simulink model "UpdatedIRECModel"  (R2025b)
settings: Solver=VariableStepAuto  StartTime=0.0  StopTime=65  MaxStep=0.001  RelTol=1e-3
model workspace (MAT data in the model file):
  bca = Simulink.Parameter
  bca.Value = [1 2]
  bca.Complexity = 'real'
  bca.Dimensions = [1 2]
  bca.DataType = 'auto'
  brakeAngle = Simulink.Parameter
  brakeAngle.Complexity = 'real'
  brakeAngle.Dimensions = [0 0]
  brakeAngle.DataType = 'auto'
undefined symbols (not defined in the file or in its folder): F, Light, MIL
libraries: aerolibanim x1, aerolibwind2 x1, aerolibatmos2 x1, aerolibasang x1
settings Model: PacingRate=141  Creator=noahweiss  LastModifiedBy=lawtonskaling

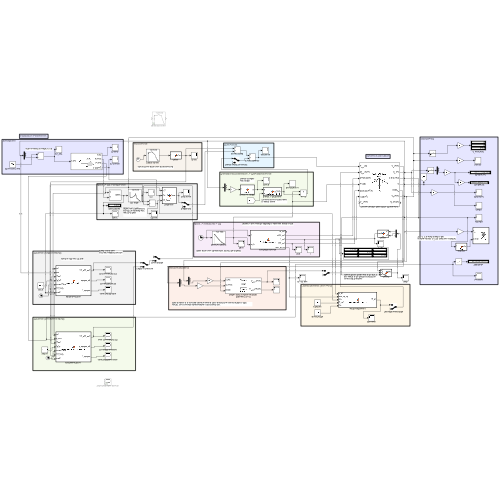
[thumbnail: Simulink's stored preview of the top-level diagram]
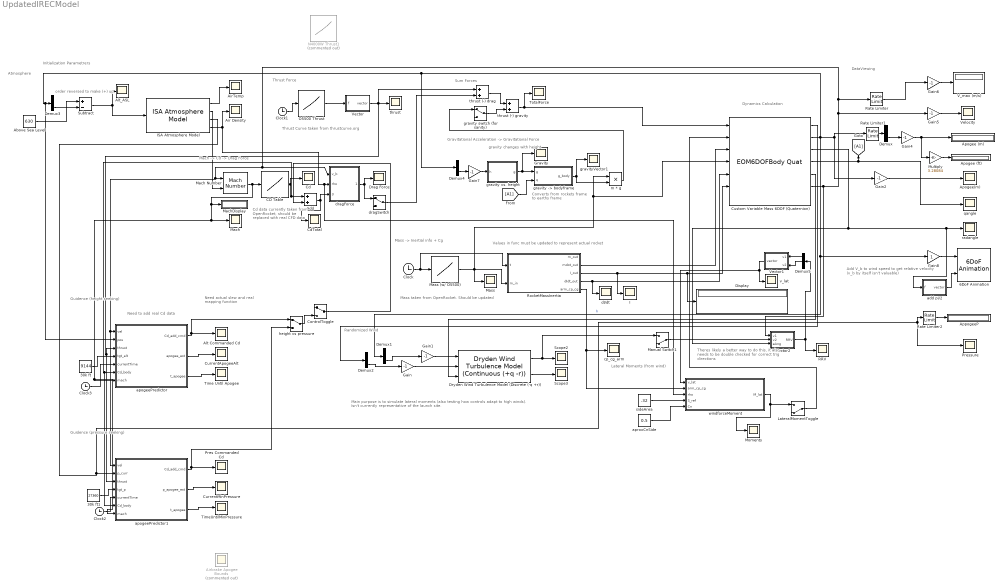
== system UpdatedIRECModel ==
  note: Theres likely a better way to do this, it also needs to be double checked for correct trig directions
  note: Need actual slew
      | and real mapping function
  note: Need to add real Cd data
  note: Guidence (height seeking)
  note: Add V_b to wind speed to get
      | relative velocity (v_b by itself isn't valuable)
  note: Values in func must be updated to represent actual rocket
  note: Lateral Moments (from wind)
  note: Main purpose is to simulate lateral moments (also testing how controls adapt to high winds). Isn't currently representative of the launch site.
  note: Randomized Wind
  note: Converts from rockets frame
      | to earths frame
  note: gravity changes
      | with height
  note: Gravitational Acceleration -> Gravitational Force
  note: Mass taken from OpenRocket. Should be updated
  note: Mass -> Inertial info + Cg
  note: Sum Forces
  note: Thrust Curve taken from thrustcurve.org
  note: Thrust Force
  note: Cd data currently
      | taken from OpenRocket, should be replaced with real CFD data
  note: Mach -> Cd -> Drag Force
  note: order reversed to make (+) up
  note: Atmosphere
  note: Initialization Parametrers
  note: Dynamics Calculation
  note: DataViewing
  note: Guidence (pressure seeking)
  30k ft : Constant  Value=9144
  30k ft1 : Constant  Value=27360
  6DoF Animation : aerolibanim/6DoF Animation  u1=[-1000 1000 -1000 1000 -10000 0]  u2=0.1  u3=200  u4=[4000 0 -5000]  u5=Fixed position  u6=[4000 -4000 -200]  u7=10  u8=off
  Above Sea Level : Constant  Value=630
  Add : Sum
  Air Density : Scope
      settings: ActiveDisplayYMinimum=0.32836250442397086  ActiveDisplayYMaximum=1.3513391175478189  DataLoggingVariableName=ScopeData2
  AirTemp : Scope
      settings: ActiveDisplayYMinimum=208.39933334266343  ActiveDisplayYMaximum=294.3971353024794  DataLoggingVariableName=ScopeData5
  "Airbrake Apogee Bounds " : Scope  Commented=on  NumInputPorts=3
      settings: DataLoggingVariableName=ScopeData31
  Alt Commanded Cd : Scope
      settings: ActiveDisplayYMinimum=-0.21249999999999994  ActiveDisplayYMaximum=1.9124999999999999  DataLoggingVariableName=ScopeData23
  Alt_ASL : Scope
      settings: ActiveDisplayYMinimum=-1  ActiveDisplayYMaximum=1  DataLoggingVariableName=ScopeData15
  Apogee (ft) : Display
  Apogee (m) : Display
      settings: Decimation=4
  Apogee(m) : Scope
      settings: ActiveDisplayYMinimum=-3110.5103645307609  ActiveDisplayYMaximum=11354.709569858003
  AppogeeP : Display
      settings: Decimation=4
  CD Table : Lookup_n-D  NumberOfTableDimensions=1  BreakpointsForDimension1=[0.007, 0.008, 0.01, 0.013, 0.017, 0.024, 0.03, 0.033, 0.037, 0.042, 0.048, 0.051, 0.056, 0.061, 0.067, 0.074, 0.08, 0.086, 0.092, 0.098, 0.102, 0.108, 0.114, 0.12, 0.126, 0.132, 0.138, 0.147, 0.161, 0.182, 0.198, 0.221, 0.248, 0.282, 0.316, 0.34, 0.375, 0.41, 0.432, 0.465, 0.502, 0.538, 0.575, 0.612, 0.647, 0.685, 0.723, 0.76, 0.798, 0.837, 0.858, 0.89, 0.929, 0.968, 1.007, 1.033, 1.071, 1.103, 1.141, 1.149, 1.16, 1.177, 1.182, 1.188, 1.197, 1.206, 1.219, 1.238, 1.257, 1.285, 1.32, 1.356, 1.368, 1.386, 1.413, 1.447, 1.48, 1.504, 1.536, 1.569, 1.601, 1.632, 1.664, 1.695, 1.725, 1.727, 1.73, 1.734, 1.74, 1.75, 1.763, 1.784, 1.793, 1.806, 1.826, 1.852, 1.876, 1.897, 1.917, 1.934, 1.937, 1.942, 1.95, 1.961, 1.969, 1.979, 1.992, 1.999, 2.008, 2.018, 2.026, 2.029, 2.033, 2.037, 2.038, 2.039, 2.041, 2.042, 2.044, 2.045, 2.046]  Table=[0.463, 0.452, 0.425, 0.409, 0.389, 0.367, 0.354, 0.348, 0.341, 0.339, 0.339, 0.339, 0.339, 0.339, 0.339, 0.339, 0.339, 0.339, 0.339, 0.339, 0.339, 0.34, 0.34, 0.34, 0.34, 0.34, 0.34, 0.34, 0.34, 0.34, 0.34, 0.341, 0.341, 0.342, 0.342, 0.343, 0.344, 0.344, 0.345, 0.346, 0.347, 0.349, 0.35, 0.352, 0.354, 0.356, 0.359, 0.362, 0.366, 0.372, 0.375, 0.383, 0.382, 0.377, 0.381, 0.408, 0.427, 0.426, 0.413, 0.409, 0.403, 0.392, 0.389, 0.385, 0.379, 0.373, 0.364, 0.352, 0.342, 0.331, 0.325, 0.321, 0.32, 0.318, 0.315, 0.311, 0.307, 0.305, 0.301, 0.298, 0.294, 0.291, 0.288, 0.285, 0.282, 0.281, 0.281, 0.281, 0.28, 0.279, 0.278, 0.276, 0.275, 0.274, 0.272, 0.269, 0.267, 0.265, 0.263, 0.262, 0.262, 0.261, 0.26, 0.259, 0.259, 0.258, 0.257, 0.256, 0.255, 0.254, 0.254, 0.253, 0.253, 0.253, 0.253, 0.252, 0.252, 0.252, 0.252, 0.252, 0.252]  InternalRulePriority=Speed  RndMeth=Simplest
  Cd : Scope
      settings: ActiveDisplayYMinimum=-0.14855998025047912  ActiveDisplayYMaximum=1.8026279606623583  DataLoggingVariableName=ScopeData8
  CdTotal : Scope
      settings: ActiveDisplayYMinimum=-0.16752402901527019  ActiveDisplayYMaximum=2.158206654782723  DataLoggingVariableName=ScopeData20
  Clock{,1..3} (4 alike) : Clock
  ControlToggle : ManualSwitch
  CurrentApogeeAlt : Scope
      settings: ActiveDisplayYMinimum=-1288.6434664799376  ActiveDisplayYMaximum=11597.791198319441  DataLoggingVariableName=ScopeData24
  CurrentMinPressure : Scope
      settings: ActiveDisplayYMinimum=22558.660012318163  ActiveDisplayYMaximum=101918.03026412864  DataLoggingVariableName=ScopeData22
  Custom Variable Mass 6DOF (Quaternion) : EOM6DOFBodyQuat  mtype=Custom Variable  vre_flag=on
  Demux{,1..5} (6 alike) : Demux  Outputs=3
  Display : Display
  Drag Force : Scope
      settings: ActiveDisplayYMinimum=-997.38496868055154  ActiveDisplayYMaximum=2083.9665587051204  DataLoggingVariableName=ScopeData3
  Dryden Wind Turbulence Model (Discrete (-q +r)) : aerolibwind2/Dryden Wind Turbulence Model  (Continuous (+q -r))  units=Metric (MKS)  spec=MIL-F-8785C  model=Discrete Dryden (+q +r)  W20=5  Wdeg=0  TurbProb=10^-2 - Light  L_high=533.4  Wingspan=1  ts=0.1  Seed=[23341 23342 23343 23345]  T_on=on
      settings: LibrarySourceBlock=|
      | aerolibwind2/Dryden Wind Turbulence Model
      | (Discrete (-q +r))
  Gain{,1..2,4..7} (7 alike) : Gain  Gain=-1
  Gain8 : Gain
  Gravity : Scope
      settings: ActiveDisplayYMinimum=9.68035453491508  ActiveDisplayYMaximum=9.8834339095755688  DataLoggingVariableName=ScopeData9
  I : Scope
      settings: ActiveDisplayYMinimum=-2.0972210212356206  ActiveDisplayYMaximum=8.771099345696328  DataLoggingVariableName=ScopeData12
  ISA Atmosphere Model : aerolibatmos2/ISA Atmosphere Model  useExtended=off  action=None  custom=off  viscosityOut=off  g=9.80665  gamma=1.4  R=287.0531  L=0.0065  h_trop=11000  h_strat=20000  rho0=1.225  P0=101325  T0=288.15  h0=0  S=110.4  Tref=273.15  muref=1.716e-5
  LateralMomentToggle : ManualSwitch  CurrentSetting=0
  Mach : Scope
      settings: ActiveDisplayYMinimum=-0.28015884352453835  ActiveDisplayYMaximum=2.052851576354866  DataLoggingVariableName=ScopeData4
  Mach Number : aerolibasang/Mach Number
  MachDisplay : Display
  Manual Switch1 : ManualSwitch  CurrentSetting=0
  Mass : Scope
      settings: ActiveDisplayYMinimum=17.378289742266098  ActiveDisplayYMaximum=34.057183726794406  DataLoggingVariableName=ScopeData7
  Mass (w/ O5500) : Lookup_n-D  NumberOfTableDimensions=1  BreakpointsForDimension1=[0, 0.009, 0.019, 0.029, 0.039, 0.044, 0.051, 0.063, 0.073, 0.078, 0.086, 0.094, 0.104, 0.109, 0.117, 0.125, 0.135, 0.147, 0.157, 0.167, 0.177, 0.187, 0.194, 0.204, 0.214, 0.224, 0.234, 0.244, 0.254, 0.269, 0.292, 0.325, 0.35, 0.387, 0.428, 0.478, 0.528, 0.563, 0.613, 0.663, 0.694, 0.74, 0.79, 0.84, 0.891, 0.941, 0.988, 1.038, 1.088, 1.138, 1.188, 1.238, 1.266, 1.308, 1.358, 1.408, 1.458, 1.491, 1.541, 1.581, 1.631, 1.641, 1.656, 1.679, 1.684, 1.692, 1.705, 1.716, 1.733, 1.759, 1.784, 1.822, 1.871, 1.921, 1.938, 1.964, 2.003, 2.053, 2.103, 2.138, 2.188, 2.238, 2.288, 2.338, 2.388, 2.438, 2.488, 2.491, 2.496, 2.502, 2.512, 2.528, 2.55, 2.585, 2.6, 2.623, 2.658, 2.708, 2.758, 2.808, 2.858, 2.908, 2.919, 2.935, 2.96, 2.997, 3.022, 3.06, 3.11, 3.138, 3.181, 3.231, 3.281, 3.3, 3.329, 3.373, 3.388, 3.41, 3.441, 3.487, 3.537, 3.544, 3.555, 3.571, 3.595, 3.609, 3.629, 3.66, 3.688, 3.73, 3.778, 3.819]  BreakpointsForDimension1FirstPoint=0  BreakpointsForDimension1Spacing=.05  Table=[31.41, 31.41, 31.39, 31.38, 31.36, 31.35, 31.33, 31.29, 31.26, 31.25, 31.22, 31.2, 31.17, 31.15, 31.13, 31.1, 31.07, 31.04, 31.01, 30.98, 30.95, 30.92, 30.9, 30.86, 30.83, 30.8, 30.77, 30.74, 30.71, 30.67, 30.6, 30.5, 30.42, 30.3, 30.17, 30.01, 29.84, 29.73, 29.56, 29.39, 29.29, 29.13, 28.96, 28.79, 28.62, 28.45, 28.28, 28.11, 27.93, 27.76, 27.59, 27.41, 27.32, 27.17, 26.99, 26.82, 26.64, 26.53, 26.35, 26.21, 26.04, 26.0, 25.95, 25.87, 25.85, 25.83, 25.79, 25.75, 25.69, 25.6, 25.52, 25.4, 25.24, 25.08, 25.03, 24.95, 24.83, 24.68, 24.53, 24.43, 24.29, 24.15, 24.01, 23.87, 23.73, 23.59, 23.45, 23.44, 23.43, 23.41, 23.38, 23.34, 23.28, 23.19, 23.15, 23.1, 23.03, 22.92, 22.82, 22.71, 22.61, 22.5, 22.48, 22.45, 22.41, 22.35, 22.32, 22.26, 22.19, 22.15, 22.1, 22.04, 21.98, 21.96, 21.93, 21.89, 21.88, 21.86, 21.84, 21.81, 21.78, 21.77, 21.77, 21.76, 21.74, 21.73, 21.72, 21.71, 21.69, 21.68, 21.66, 21.65]  ExtrapMethod=Clip  UseLastTableValue=on  InternalRulePriority=Speed  RndMeth=Simplest  SupportTunableSize=on
  Moments : Scope
      settings: ActiveDisplayYMinimum=-0.037322938130257846  ActiveDisplayYMaximum=0.019814293763566297  DataLoggingVariableName=ScopeData19
  Multiply : Gain  Gain=3.28084
  N4000W Thrust1 : Lookup_n-D  Commented=on  NumberOfTableDimensions=1  BreakpointsForDimension1=[0.01;0.029;0.03;0.031;0.039;0.049;0.05;0.06;0.07000000000000001;0.078;0.08799999999999999;0.12;0.148;0.247;0.398;0.577;0.774;0.964;1.172;1.341;1.51;1.661;1.837;2.027;2.157;2.295;2.336;2.505;2.633;2.794;2.97;3.131;3.3;3.449;3.547;3.607;3.708;3.825;3.927;4.054;4.205;4.314;4.394;4.462;4.511;4.631;4.761;4.854;4.906]  Table=[39.369999999999997;393.70100000000002;1742.126;2209.6460000000002;2874.0160000000001;2534.4490000000001;3469.4879999999998;3809.0549999999998;4079.7240000000002;4242.1260000000002;4384.8429999999998;4330.7089999999998;4227.3620000000001;4242.1260000000002;4296.2600000000002;4350.3940000000002;4438.9759999999997;4512.7950000000001;4566.9290000000001;4621.0630000000001;4621.0630000000001;4655.5119999999997;4675.1970000000001;4709.6459999999997;4729.3310000000001;4749.0159999999996;4749.0159999999996;4694.8819999999996;4655.5119999999997;4547.2439999999997;4478.3459999999995;4384.8429999999998;4315.9449999999997;4261.8109999999997;4261.8109999999997;4207.6769999999997;3720.4720000000002;2893.701;2445.866;2155.5120000000002;1850.394;1471.4570000000001;1097.441;841.53499999999997;698.81899999999996;521.654;265.74799999999999;123.03100000000001;0]  ExtrapMethod=Clip  UseLastTableValue=on  InternalRulePriority=Speed  RndMeth=Simplest
  O5500 Thrust : Lookup_n-D  NumberOfTableDimensions=1  BreakpointsForDimension1=[0.009, 0.044, 0.063, 0.078, 0.094, 0.109, 0.125, 0.147, 0.194, 0.35, 0.428, 0.563, 0.694, 0.988, 1.266, 1.491, 1.581, 1.641, 1.684, 1.716, 1.784, 1.938, 2.138, 2.491, 2.6, 2.919, 3.022, 3.138, 3.3, 3.388, 3.441, 3.544, 3.609, 3.688, 3.778, 3.819, 3.853, 3.897, 3.981, 3.997]  Table=[20.408, 7112.245, 6734.694, 6897.959, 6612.245, 6765.306, 6540.816, 6581.633, 6520.408, 6795.918, 7091.837, 7285.714, 7408.163, 7581.633, 7622.449, 7724.49, 7653.061, 7540.816, 7500.0, 7336.735, 7224.49, 6785.714, 6326.531, 5897.959, 5704.082, 3540.816, 3408.163, 2887.755, 2234.694, 1673.469, 1489.796, 1418.367, 1295.918, 816.327, 653.061, 581.633, 489.796, 285.714, 20.408, 0.0]  ExtrapMethod=Clip  UseLastTableValue=on  InternalRulePriority=Speed  RndMeth=Simplest
  Pres Commanded Cd : Scope
      settings: ActiveDisplayYMinimum=-0.13333983055562462  ActiveDisplayYMaximum=1.2000584750006218  DataLoggingVariableName=ScopeData27
  Pressure : Scope
      settings: ActiveDisplayYMinimum=27434.677675772422  ActiveDisplayYMaximum=27734.888035030621  DataLoggingVariableName=ScopeData28
  RRV : Scope
      settings: ActiveDisplayYMinimum=-147.82773037596519  ActiveDisplayYMaximum=87.725846488197178  DataLoggingVariableName=ScopeData30
  Rate Limiter : RateLimiter  RisingSlewLimit=0  FallingSlewLimit=-99999  SampleTimeMode=inherited
  Rate Limiter1 : RateLimiter  RisingSlewLimit=0  FallingSlewLimit=-99999  SampleTimeMode=inherited
  Rate Limiter2 : RateLimiter  RisingSlewLimit=0  FallingSlewLimit=-99999  SampleTimeMode=inherited
  RocketMassInertia : MATLAB Function  TreatAsAtomicUnit=on
  Scope2 : Scope
      settings: ActiveDisplayYMinimum=-3.5919608640744958  ActiveDisplayYMaximum=4.9299230789313464  DataLoggingVariableName=ScopeData10
  Scope3 : Scope
      settings: ActiveDisplayYMinimum=-6.9396586411031267E+307  ActiveDisplayYMaximum=1.2409351060971885E+307  DataLoggingVariableName=ScopeData13
  Subtract : Sum  Inputs=+-
  Time Until Apogee : Scope
      settings: ActiveDisplayYMinimum=-142.04754177762925  ActiveDisplayYMaximum=334.02527575200287  DataLoggingVariableName=ScopeData25
  "TimeUntilMinPressure " : Scope
      settings: ActiveDisplayYMinimum=-169.43788860496815  ActiveDisplayYMaximum=400.46442472293245  DataLoggingVariableName=ScopeData26
  TotalForce : Scope
      settings: ActiveDisplayYMinimum=-1336.7372091363745  ActiveDisplayYMaximum=2383.8615158167772  DataLoggingVariableName=ScopeData6
  V_max (m/s) : Display
  Vector : MATLAB Function  TreatAsAtomicUnit=on
  Vector1 : MATLAB Function  TreatAsAtomicUnit=on
  Vector2 : MATLAB Function  TreatAsAtomicUnit=on
  Velocity : Scope
      settings: ActiveDisplayYMinimum=-269.31086851436129  ActiveDisplayYMaximum=736.30958702242276
  add pi/2 : MATLAB Function  TreatAsAtomicUnit=on
  apogeePredictor : MATLAB Function  TreatAsAtomicUnit=on
  apogeePredictor1 : MATLAB Function  TreatAsAtomicUnit=on
  aproxCnSide : Constant  Value=0.5
  cp_cg_arm : Scope
      settings: ActiveDisplayYMinimum=-0.50903350176661866  ActiveDisplayYMaximum=0.54777232101906159  DataLoggingVariableName=ScopeData21
  dI/dt : Scope
      settings: ActiveDisplayYMinimum=-1  ActiveDisplayYMaximum=1  DataLoggingVariableName=ScopeData11
  dragForce : MATLAB Function  TreatAsAtomicUnit=on
  dragSwitch : ManualSwitch
  "gravity -> bodyframe" : MATLAB Function  TreatAsAtomicUnit=on
  gravity switch (for sanity) : ManualSwitch
  gravity vs. height : MATLAB Function  TreatAsAtomicUnit=on
  gravityVector1 : Scope
      settings: ActiveDisplayYMinimum=-243.141573178529  ActiveDisplayYMaximum=145.53469052356505  DataLoggingVariableName=ScopeData17
  height vs pressure : ManualSwitch
  m * g : Product
  qangle : Scope
      settings: ActiveDisplayYMinimum=-0.69920344245396326  ActiveDisplayYMaximum=1.5743399638672304  DataLoggingVariableName=ScopeData18
  radangle : Scope
      settings: ActiveDisplayYMinimum=-3.9268979901815744  ActiveDisplayYMaximum=3.926971640420561  DataLoggingVariableName=ScopeData16
  sideArea : Constant  Value=.32
  thrust : Scope
      settings: ActiveDisplayYMinimum=-6112.1844862335238  ActiveDisplayYMaximum=743.283877041516  DataLoggingVariableName=ScopeData14
  thrust (-) drag : Sum
  thrust (-) gravity : Sum
  v_lat : Scope
      settings: ActiveDisplayYMinimum=-11.656849883026286  ActiveDisplayYMaximum=6.4269462139654019  DataLoggingVariableName=ScopeData29
  windforceMoment : MATLAB Function  TreatAsAtomicUnit=on
  wires:
  Custom Variable Mass 6DOF (Quaternion)/6 -> Vector2/1(v1), dragForce/1(v_b), apogeePredictor1/1(vel), apogeePredictor/1(vel), Mach Number/1, Rate Limiter/1, Gain5/1
  Rate Limiter/1 -> Gain6/1
  ISA Atmosphere Model/4 -> windforceMoment/3(rho), dragForce/2(rho), Air Density/1
  Rate Limiter1/1 -> Demux/1
  Demux/3 -> Gain4/1
  dragForce/1(drag_force) -> Drag Force/1, dragSwitch/1
  CD Table/1 -> apogeePredictor1/6(Cd_body), apogeePredictor/6(Cd_body), Add/1, Cd/1
  ISA Atmosphere Model/1 -> AirTemp/1
  Clock1/1 -> O5500 Thrust/1
  O5500 Thrust/1 -> Vector/1(f)
  Vector/1(vector) -> thrust (-) drag/1, apogeePredictor1/3(thrust), apogeePredictor/3(thrust), thrust/1
  dragSwitch/1 -> thrust (-) drag/2
  RocketMassInertia/4(dIdt_out) -> Custom Variable Mass 6DOF (Quaternion)/5, dI/dt/1
  RocketMassInertia/3(I_out) -> I/1, Custom Variable Mass 6DOF (Quaternion)/6, Display/1
  Mass (w/ O5500)/1 -> RocketMassInertia/2(m_in), Custom Variable Mass 6DOF (Quaternion)/4, m * g/1, Mass/1
  thrust (-) drag/1 -> thrust (-) gravity/1
  thrust (-) gravity/1 -> Custom Variable Mass 6DOF (Quaternion)/1, TotalForce/1
  m * g/1 -> gravity switch (for sanity)/1
  gravity switch (for sanity)/1 -> thrust (-) gravity/2
  Above Sea Level/1 -> Subtract/1
  Custom Variable Mass 6DOF (Quaternion)/2 -> Gain2/1, Rate Limiter1/1, Gain8/1, Demux1/1, Demux4/1, apogeePredictor/2(pos), Demux3/1  "h"
  "gravity -> bodyframe"/1(g_body) -> gravityVector1/1, m * g/2
  Custom Variable Mass 6DOF (Quaternion)/5 -> Dryden Wind Turbulence Model (Discrete (-q +r))/3
  Dryden Wind Turbulence Model (Discrete (-q +r))/1 -> Scope2/1, Manual Switch1/1
  Dryden Wind Turbulence Model (Discrete (-q +r))/2 -> Scope3/1
  Demux1/3 -> Gain1/1
  Demux2/3 -> Gain/1
  Custom Variable Mass 6DOF (Quaternion)/1 -> Demux2/1
  Gain/1 -> Dryden Wind Turbulence Model (Discrete (-q +r))/2
  Gain1/1 -> Dryden Wind Turbulence Model (Discrete (-q +r))/1
  RocketMassInertia/2(mdot_out) -> Custom Variable Mass 6DOF (Quaternion)/3
  Custom Variable Mass 6DOF (Quaternion)/3 -> add pi/2/1(f), radangle/1, Vector2/3(eAng)
  Manual Switch1/1 -> Vector2/2(v2)
  Demux3/3 -> Subtract/2
  Subtract/1 -> ISA Atmosphere Model/1, Alt_ASL/1
  ISA Atmosphere Model/2 -> Mach Number/2
  Mach Number/1 -> Mach/1, apogeePredictor1/7(mach), apogeePredictor/7(mach), MachDisplay/1, CD Table/1
  Gain2/1 -> Apogee(m)/1
  Gain5/1 -> Velocity/1
  Gain6/1 -> V_max (m/s)/1
  Gain4/1 -> Multiply/1, Apogee (m)/1
  gravity vs. height/1(g) -> Gravity/1, "gravity -> bodyframe"/1(g)
  Gain7/1 -> gravity vs. height/1(h)
  Demux4/3 -> Gain7/1
  Custom Variable Mass 6DOF (Quaternion)/4 -> qangle/1, [A1]
  aproxCnSide/1 -> windforceMoment/5(Cn)
  LateralMomentToggle/1 -> Custom Variable Mass 6DOF (Quaternion)/2
  sideArea/1 -> windforceMoment/4(S_ref)
  Gain8/1 -> 6DoF Animation/1
  [A1] -> "gravity -> bodyframe"/2(q)
  Clock/1 -> RocketMassInertia/1(t), Mass (w/ O5500)/1
  Multiply/1 -> Apogee (ft)/1
  windforceMoment/1(M_lat) -> Moments/1, LateralMomentToggle/1
  30k ft/1 -> apogeePredictor/4(tgt_alt)
  Clock3/1 -> apogeePredictor/5(currentTime)
  apogeePredictor/2(apogee_est) -> CurrentApogeeAlt/1
  apogeePredictor/3(t_apogee) -> Time Until Apogee/1
  RocketMassInertia/5(arm_cp_cg) -> windforceMoment/2(arm_cp_cg), cp_cg_arm/1
  apogeePredictor/1(Cd_add_cmd) -> height vs pressure/1, Alt Commanded Cd/1
  Add/1 -> CdTotal/1, dragForce/3(Cd_base)
  ControlToggle/1 -> Add/2
  add pi/2/1(vector) -> 6DoF Animation/2
  apogeePredictor1/3(t_apogee) -> "TimeUntilMinPressure "/1
  apogeePredictor1/1(Cd_add_cmd) -> height vs pressure/2, Pres Commanded Cd/1
  apogeePredictor1/2(p_apogee_est) -> CurrentMinPressure/1
  30k ft1/1 -> apogeePredictor1/4(tgt_p)
  Clock2/1 -> apogeePredictor1/5(currentTime)
  height vs pressure/1 -> ControlToggle/2
  ISA Atmosphere Model/3 -> Rate Limiter2/1, Pressure/1, apogeePredictor1/2(p_curr)
  Rate Limiter2/1 -> AppogeeP/1
  Vector1/1(vector) -> windforceMoment/1(v_lat), v_lat/1
  Demux5/1 -> Vector1/1(v1)
  Demux5/2 -> Vector1/2(v2)
  Vector2/1(RRV) -> RRV/1, Demux5/1

== matlab function UpdatedIRECModel/Vector1 ==
  data: v1 input; v2 input; vector output
function vector = fcn(v1, v2)

vector = zeros(1,3);
vector(1) = v1;
vector(2) = v2;

end

== matlab function UpdatedIRECModel/Vector2 ==
  data: v1 input; v2 input; RRV output; eAng input
function RRV = fcn(v1, v2, eAng)

RRV = zeros(1,3);
RRV(1) = v1(1) + cos(eAng(1)) * v2(1);
RRV(2) = v1(2) + cos(eAng(2)) * v2(2);
RRV(3) = v1(3) + cos(eAng(3)) * v2(3);

end

== matlab function UpdatedIRECModel/RocketMassInertia ==
  settings: updateMethod=DISCRETE
  data: t input; m_out output; mdot_out output; I_out output; dIdt_out output; m_in input; arm_cp_cg output
function [m_out, mdot_out, I_out, dIdt_out, arm_cp_cg] = RocketMassInertia(t, m_in)

persistent m0_total m_prop0

D_body   = 0.1016;
R_body   = D_body/2;

L_total  = 2.40;
L_nose   = 0.45;
L_body   = L_total - L_nose;

L_motor     = 0.65;
x_motor_fwd = L_total - L_motor;
x_motor_aft = L_total;

x_nose_cg   = 0.27 * L_nose;
x_tube_cg   = L_nose + 0.5 * L_body;
x_avionics  = L_nose + 0.15;
x_airbrake  = L_nose + 0.90;
x_fins      = L_total - 0.05;
x_case      = x_motor_fwd + 0.5 * L_motor;
x_other     = x_avionics;

m_nose     = 0.8;
m_tube     = 1.2;
m_avionics = 0.7;
m_airbrake = 0.5;
m_case     = 1.0;
m_fins     = 0.6;
m_other    = 0.4;

m_struct_total = m_nose + m_tube + m_avionics + m_airbrake + m_case + m_fins + m_other;

R_prop  = 0.035;

if isempty(m0_total)
    m0_total = m_in;
    m_prop0  = max(m0_total - m_struct_total, 0);
end

m_total = m_in;
if m_total < m_struct_total
    m_total = m_struct_total;
end

m_prop = m_total - m_struct_total;
if m_prop < 0
    m_prop = 0;
end
if m_prop > m_prop0
    m_prop = m_prop0;
end

x_prop_cg = x_case;
L_prop    = L_motor;

Ixx_tube_cg = 0.5 * m_tube * R_body^2;
Iyy_tube_cg = m_tube * (L_body^2 / 12 + R_body^2 / 4);
Izz_tube_cg = Iyy_tube_cg;

if m_prop > 0
    Ixx_prop_cg = 0.5 * m_prop * R_prop^2;
    Iyy_prop_cg = m_prop * (L_prop^2 / 12 + R_prop^2 / 4);
    Izz_prop_cg = Iyy_prop_cg;
else
    Ixx_prop_cg = 0;
    Iyy_prop_cg = 0;
    Izz_prop_cg = 0;
end

Ixx_case_cg = 0.5 * m_case * R_prop^2;
Iyy_case_cg = m_case * (L_motor^2 / 12 + R_prop^2 / 4);
Izz_case_cg = Iyy_case_cg;

m_total_components = m_struct_total + m_prop;

if m_total_components <= 0
    x_cg = x_tube_cg;
else
    x_cg = (m_nose * x_nose_cg + m_tube * x_tube_cg + m_avionics * x_avionics + ...
            m_airbrake * x_airbrake + m_case * x_case + m_fins * x_fins + ...
            m_other * x_other + m_prop * x_prop_cg) / m_total_components;
end

dx_tube  = x_tube_cg   - x_cg;
dx_case  = x_case      - x_cg;
dx_prop  = x_prop_cg   - x_cg;
dx_nose  = x_nose_cg   - x_cg;
dx_av    = x_avionics  - x_cg;
dx_ab    = x_airbrake  - x_cg;
dx_fin   = x_fins      - x_cg;
dx_other = x_other     - x_cg;

Ixx_tube = Ixx_tube_cg;
Iyy_tube = Iyy_tube_cg + m_tube     * dx_tube^2;
Izz_tube = Izz_tube_cg + m_tube     * dx_tube^2;

Ixx_case = Ixx_case_cg;
Iyy_case = Iyy_case_cg + m_case     * dx_case^2;
Izz_case = Izz_case_cg + m_case     * dx_case^2;

Ixx_prop = Ixx_prop_cg;
Iyy_prop = Iyy_prop_cg + m_prop     * dx_prop^2;
Izz_prop = Izz_prop_cg + m_prop     * dx_prop^2;

Ixx_nose = 0;
Iyy_nose = m_nose     * dx_nose^2;
Izz_nose = m_nose     * dx_nose^2;

Ixx_av   = 0;
Iyy_av   = m_avionics * dx_av^2;
Izz_av   = m_avionics * dx_av^2;

Ixx_ab   = 0;
Iyy_ab   = m_airbrake * dx_ab^2;
Izz_ab   = m_airbrake * dx_ab^2;

Ixx_fin  = 0;
Iyy_fin  = m_fins     * dx_fin^2;
Izz_fin  = m_fins     * dx_fin^2;

Ixx_other = 0;
Iyy_other = m_other   * dx_other^2;
Izz_other = m_other   * dx_other^2;

Ixx = Ixx_tube + Ixx_case + Ixx_prop + Ixx_nose + Ixx_av + Ixx_ab + Ixx_fin + Ixx_other;
Iyy = Iyy_tube + Iyy_case + Iyy_prop + Iyy_nose + Iyy_av + Iyy_ab + Iyy_fin + Iyy_other;
Izz = Izz_tube + Izz_case + Izz_prop + Izz_nose + Izz_av + Izz_ab + Izz_fin + Izz_other;

% kill roll coupling: make Iyy = Izz
I_perp = 0.5 * (Iyy + Izz);
Iyy    = I_perp;
Izz    = I_perp;

I_mat = zeros(3,3);
I_mat(1,1) = Ixx;
I_mat(2,2) = Iyy;
I_mat(3,3) = Izz;

m_out    = m_total;
I_out    = I_mat;
dIdt_out = zeros(3,3);
mdot_out = 0;

x_cp = 1.8; % [m] CP from nose (tune this)
arm_cp_cg = x_cp - x_cg;
end

== matlab function UpdatedIRECModel/dragForce ==
  data: v_b input; drag_force output; rho input; Cd_base input
function drag_force = fcn(v_b, rho, Cd_base)

    D = 0.15672;
    R = D/2;
    A_ref = pi * R^2;

    if ~isfinite(rho) || rho <= 0 || ~isfinite(Cd_base) || Cd_base <= 0
        drag_force = zeros(3,1);
        return;
    end

    vx = v_b(1); vy = v_b(2); vz = v_b(3);
    v2 = vx*vx + vy*vy + vz*vz;
    if v2 < 1e-8
        drag_force = zeros(3,1);
        return;
    end

    V = sqrt(v2);
    q = 0.5 * rho * v2;

    % angle of attack relative to body x
    alpha = atan2(sqrt(vy*vy + vz*vz), vx);

    % constrict AoA
    alpha_max = deg2rad(5);       % 5 deg cap
    if alpha > alpha_max
        alpha = alpha_max;
    end

    k_alpha = 0.5;                 % tweak 0–1 range
    Cd_eff = Cd_base + k_alpha * (alpha * alpha);

    Dmag = q * Cd_eff * A_ref;

    drag_force = -(Dmag / V) * v_b;
end

== matlab function UpdatedIRECModel/gravity vs. height ==
  data: h input; g output
function g = gravity(h)

G = 6.674e-11;
M = 5.972e24;
R = 6.371e6;

g = G * M ./ (R + h).^2;
end

== matlab function UpdatedIRECModel/add pi//2 ==
  data: f input; vector output
function vector = fcn(f)
f = f(:);
vector = f;
vector(2) = f(2) + pi/2;
end

== matlab function UpdatedIRECModel/windforceMoment ==
  data: v_lat input; M_lat output; arm_cp_cg input; rho input; S_ref input; Cn input
function M_lat = lateralAeroMoments(v_lat, arm_cp_cg, rho, S_ref, Cn)
   Vx = v_lat(1);
   Vy = v_lat(2);

   if ~isfinite(Vx) || ~isfinite(Vy) || ~isfinite(arm_cp_cg) || ~isfinite(rho) || ~isfinite(S_ref) || ~isfinite(Cn)
        M_lat = [0; 0; 0];
        return;
   end
    
   V_lat = sqrt(Vx*Vx + Vy*Vy);
   q_dyn = 0.5 * rho * (Vx*Vx + Vy*Vy);
   Fn = q_dyn * S_ref * Cn;

   Fx = -Fn * (Vx / V_lat);
   Fy = -Fn * (Vy / V_lat);

   Mx = abs(arm_cp_cg) * Fx;
   My = abs(arm_cp_cg) * Fy;

   M_lat = [Mx; My; 0];

end

== matlab function UpdatedIRECModel/gravity -> bodyframe ==
  data: g input; g_body output; q input
function g_body = gravityBodyQuat(g, q)

q0 = q(1);
q1 = q(2);
q2 = q(3);
q3 = q(4);

% Direction Cosine Matrix: inertial -> body
R = [ 1-2*(q2^2+q3^2),   2*(q1*q2+q0*q3),   2*(q1*q3-q0*q2);
      2*(q1*q2-q0*q3),   1-2*(q1^2+q3^2),   2*(q2*q3+q0*q1);
      2*(q1*q3+q0*q2),   2*(q2*q3-q0*q1),   1-2*(q1^2+q2^2) ];

% Gravity direction in inertial frame (NED)
g_inertial = [0; 0; g];   % +Z = down

% Transform to BODY frame
g_body = R * g_inertial;
end

== matlab function UpdatedIRECModel/Vector ==
  data: f input; vector output
function vector = fcn(f)

vector = zeros(3,1);
vector(3) = -f;

end

== matlab function UpdatedIRECModel/apogeePredictor ==
  settings: updateMethod=DISCRETE
  data: vel input; pos input; thrust input; Cd_add_cmd output; tgt_alt input; currentTime input; apogee_est output; t_apogee output; Cd_body input; mach input
function [Cd_add_cmd, apogee_est, t_apogee] = apogeePredictor(vel, pos, thrust, tgt_alt, currentTime, Cd_body, mach)
    % --- Configuration and Physical Constants ---
    persistent Cd_add_prev t_prev apogee_time prev_vel_up
    m = 18.9;                       % Rocket mass (kg)
    A = 8107/(1000^2);              % Reference area (m^2)
    A_over_m = A/m;
    g0 = 9.80665;                   % Standard gravity
    Re = 6371000;                   % Earth radius
    Cd_body_nominal = 0.7;          % Default dry rocket drag coefficient
    Cd_total_max = 1.7;             % Maximum drag with airbrakes fully deployed
    
    % --- Input Validation and Bounds Handling ---
    if nargin < 6 || isempty(Cd_body)
        Cd_body = Cd_body_nominal;
    end
    if nargin < 7 || isempty(mach)
        mach = 0;
    end
    Cd_body = max(0, Cd_body);
    Cd_air_min = 0;
    Cd_air_max = max(0, Cd_total_max - Cd_body); % Max allowable drag from airbrakes
    
    % --- Control Parameters ---
    burn_window = 3.0;              % Time window for motor burn
    thrust_thresh = 1.0;            % Newton threshold for motor activity
    alt_tol = 0.0;                  % Target altitude tolerance
    max_iter = 12;                  % Iterations for binary search of Cd
    max_rate = 1.5;                 % Max slew rate (Cd change per second)

    % --- Persistent State Initialization ---
    if isempty(Cd_add_prev)
        Cd_add_prev = 0;
    end
    if isempty(t_prev)
        t_prev = currentTime;
    end
    if isempty(apogee_time)
        apogee_time = NaN;
    end
    if isempty(prev_vel_up)
        prev_vel_up = 0;
    end
    
    % --- Timing and Delta-T Calculation ---
    dt_cmd = currentTime - t_prev;
    if dt_cmd <= 0
        dt_cmd = 0.02;
    elseif dt_cmd > 0.1
        dt_cmd = 0.1;
    end
    t_prev = currentTime;
    Cd_add_prev = max(Cd_air_min, min(Cd_air_max, Cd_add_prev));
    
    % --- Coordinate System Mapping ---
    % Identifies the vertical axis based on the largest positional component (assuming ENU/NED)
    if numel(pos) >= 3
        [~, idx] = max([abs(pos(2)), abs(pos(3))]);
        vert_idx = idx + 1;
    else
        vert_idx = 2;
    end
    alt_up = max(0, -pos(vert_idx));  % Conversion to up-positive altitude
    vel_up = -vel(vert_idx);          % Conversion to up-positive velocity
    thrust_mag = norm(thrust);
    
    % --- Apogee Detection ---
    % Monitors for the zero-crossing of vertical velocity
    if isnan(apogee_time)
        if prev_vel_up > 0 && vel_up <= 0
            apogee_time = currentTime;
        end
    end
    prev_vel_up = vel_up;
    
    % --- Default Prediction State ---
    Cd_add_target = Cd_add_prev;  
    apogee_est = alt_up;
    t_apogee = currentTime;
    
    % --- Control Logic State Machine ---
    
    % Case 1: Recovery Phase (Post-apogee)
    if ~isnan(apogee_time) && currentTime >= apogee_time + 2
        Cd_add_target = 0; % Retract airbrakes for parachute deployment
        apogee_est = alt_up;
        t_apogee = apogee_time;
        
    % Case 2: Boost Phase
    elseif currentTime < burn_window && thrust_mag > thrust_thresh
        Cd_add_target = 0; % Brakes closed while motor is firing
        
    % Case 3: Transonic/Supersonic Logic
    elseif mach > 1
        Cd_add_target = 0; % Keep brakes closed above Mach 1 to avoid structural damage
        [apogee_est, dt_est] = simulateCoastVarCd(alt_up, vel_up, Cd_body, Cd_add_prev, Cd_add_target, max_rate, A_over_m, g0, Re);
        t_apogee = currentTime + dt_est;
        
    % Case 4: Descent or Overshoot
    elseif vel_up <= 0 || alt_up >= tgt_alt
        Cd_add_target = Cd_air_max; % Deploy fully to slow down if already past target
        [apogee_est, dt_est] = simulateCoastVarCd(alt_up, vel_up, Cd_body, Cd_add_prev, Cd_add_target, max_rate, A_over_m, g0, Re);
        t_apogee = currentTime + dt_est;
        
    % Case 5: Active Coast Control (Airbrake Modulation)
    else
        % Check if we would undershoot even with brakes fully retracted
        [ap_clean, dt_clean] = simulateCoastVarCd(alt_up, vel_up, Cd_body, Cd_add_prev, 0, max_rate, A_over_m, g0, Re);
        if ap_clean <= tgt_alt + alt_tol
            Cd_add_target = 0;
            apogee_est = ap_clean;
            t_apogee = currentTime + dt_clean;
        elseif Cd_air_max <= 0
            Cd_add_target = 0;
            apogee_est = ap_clean;
            t_apogee = currentTime + dt_clean;
        else
            % Check if we would still overshoot with brakes fully deployed
            [ap_brake, dt_brake] = simulateCoastVarCd(alt_up, vel_up, Cd_body, Cd_add_prev, Cd_air_max, max_rate, A_over_m, g0, Re);
            if ap_brake > tgt_alt
                Cd_add_target = Cd_air_max;
                apogee_est = ap_brake;
                t_apogee = currentTime + dt_brake;
            else
                % Optimization: Binary Search for the precise Cd required to hit tgt_alt
                lowAdd = 0;
                highAdd = Cd_air_max;
                lowAp = ap_clean;
                highAp = ap_brake;
                lowT = dt_clean;
                highT = dt_brake;
                Cd_add_target = Cd_add_prev;
                for k = 1:max_iter
                    midAdd = 0.5*(lowAdd + highAdd);
                    [midAp, midT] = simulateCoastVarCd(alt_up, vel_up, Cd_body, Cd_add_prev, midAdd, max_rate, A_over_m, g0, Re);
                    if abs(midAp - tgt_alt) <= alt_tol
                        Cd_add_target = midAdd;
                        apogee_est = midAp;
                        t_apogee = currentTime + midT;
                        break;
                    end
                    if midAp > tgt_alt
                        lowAdd = midAdd;
                        lowAp = midAp;
                        lowT = midT;
                    else
                        highAdd = midAdd;
                        highAp = midAp;
                        highT = midT;
                    end
                    if k == max_iter
                        Cd_add_target = 0.5*(lowAdd + highAdd);
                        [apogee_est, dt_final] = simulateCoastVarCd(alt_up, vel_up, Cd_body, Cd_add_prev, Cd_add_target, max_rate, A_over_m, g0, Re);
                        t_apogee = currentTime + dt_final;
                    end
                end
            end
        end
    end
    
    % --- Slew Rate Limiting and Command Output ---
    Cd_add_target = max(Cd_air_min, min(Cd_air_max, Cd_add_target));
    max_step = max_rate * dt_cmd;
    delta = Cd_add_target - Cd_add_prev;
    
    % Limit the change in Cd based on mechanical motor speed (max_rate)
    if delta > max_step
        delta = max_step;
    elseif delta < -max_step
        delta = -max_step;
    end
    
    Cd_add_cmd = Cd_add_prev + delta;
    Cd_add_cmd = max(Cd_air_min, min(Cd_air_max, Cd_add_cmd));
    Cd_add_prev = Cd_add_cmd;
end

function [apogee, dt_to_apogee] = simulateCoastVarCd(h0, v0, Cd_body, Cd_add_initial, Cd_add_target, max_rate, A_over_m, g0, Re)
    % --- Numerical Simulation of Coast Phase ---
    if v0 <= 0
        apogee = max(0, h0);
        dt_to_apogee = 0;
        return;
    end
    h = h0;
    v = v0;
    t = 0;
    dt = 0.02; % Time step for integration
    max_steps = 9000;
    Cd_add_initial = max(0, Cd_add_initial);
    Cd_add_target = max(0, Cd_add_target);
    
    for step = 1:max_steps
        % Step forward using RK4 integration
        [h_next, v_next] = rk4StepVarCd(h, v, t, dt, Cd_body, Cd_add_initial, Cd_add_target, max_rate, A_over_m, g0, Re);
        
        % Check for apogee (velocity zero-crossing)
        if v > 0 && v_next <= 0
            % Interpolate to find the precise apogee point
            Cd_add_now = cdProfile(t, Cd_add_initial, Cd_add_target, max_rate);
            Cd_total_now = Cd_body + Cd_add_now;
            a0 = computeAccel(h, v, Cd_total_now, A_over_m, g0, Re);
            frac = v/(v - v_next);
            t_zero = frac*dt;
            apogee = h + v*t_zero + 0.5*a0*t_zero^2;
            apogee = max(0, apogee);
            dt_to_apogee = t + t_zero;
            return;
        end
        h = h_next;
        v = v_next;
        t = t + dt;
        if h <= 0 % Terminate if ground hit
            apogee = 0;
            dt_to_apogee = t;
            return;
        end
    end
    apogee = max(0, h);
    dt_to_apogee = t;
end

function [h_out, v_out] = rk4StepVarCd(h, v, t, dt, Cd_body, Cd_add_initial, Cd_add_target, max_rate, A_over_m, g0, Re)
    % --- Runge-Kutta 4th Order Integration Step ---
    % Evaluates physics at 4 points across the time step to maintain accuracy
    
    % k1: Start of step
    Cd_add1 = cdProfile(t, Cd_add_initial, Cd_add_target, max_rate);
    Cd_total1 = Cd_body + Cd_add1;
    k1_v = computeAccel(h, v, Cd_total1, A_over_m, g0, Re);
    k1_h = v;
    
    % k2: Midpoint
    t2 = t + 0.5*dt;
    v2 = v + 0.5*dt*k1_v;
    h2 = h + 0.5*dt*k1_h;
    Cd_add2 = cdProfile(t2, Cd_add_initial, Cd_add_target, max_rate);
    Cd_total2 = Cd_body + Cd_add2;
    k2_v = computeAccel(h2, v2, Cd_total2, A_over_m, g0, Re);
    k2_h = v2;
    
    % k3: Midpoint re-evaluation
    v3 = v + 0.5*dt*k2_v;
    h3 = h + 0.5*dt*k2_h;
    Cd_add3 = cdProfile(t2, Cd_add_initial, Cd_add_target, max_rate);
    Cd_total3 = Cd_body + Cd_add3;
    k3_v = computeAccel(h3, v3, Cd_total3, A_over_m, g0, Re);
    k3_h = v3;
    
    % k4: End of step
    t4 = t + dt;
    v4 = v + dt*k3_v;
    h4 = h + dt*k3_h;
    Cd_add4 = cdProfile(t4, Cd_add_initial, Cd_add_target, max_rate);
    Cd_total4 = Cd_body + Cd_add4;
    k4_v = computeAccel(h4, v4, Cd_total4, A_over_m, g0, Re);
    k4_h = v4;
    
    % Weighted average update
    v_out = v + (dt/6)*(k1_v + 2*k2_v + 2*k3_v + k4_v);
    h_out = h + (dt/6)*(k1_h + 2*k2_h + 2*k3_h + k4_h);
end

function Cd_add = cdProfile(t, Cd_initial, Cd_target, max_rate)
    % --- Airbrake Slew Profile ---
    % Calculates the Cd at time 't' during the simulation, accounting for mechanical speed
    delta = Cd_target - Cd_initial;
    max_delta = max_rate * t;
    if delta > 0
        delta_eff = min(delta, max_delta);
    else
        delta_eff = max(delta, -max_delta);
    end
    Cd_add = Cd_initial + delta_eff;
end

function a = computeAccel(h, v, Cd_total, A_over_m, g0, Re)
    % --- Physics: Acceleration Model ---
    rho = densityAtAlt(h, g0);
    g_eff = g0*(Re/(Re + h))^2; % Inverse-square gravity
    drag = -0.5*rho*Cd_total*A_over_m*v*abs(v); % Drag equation (opposite to velocity)
    a = drag - g_eff;
end

function rho = densityAtAlt(h, g0)
    % --- International Standard Atmosphere (ISA) Model ---
    % Calculates air density (kg/m^3) based on altitude layers
    h = max(0, h);
    R = 287.053; % Gas constant for air
    
    % Troposphere (up to 11km)
    if h <= 11000
        T = 288.15 - 0.0065*h;
        p = 101325*(T/288.15)^(g0/(R*0.0065));
        rho = p/(R*T);
    % Lower Stratosphere (11km to 20km)
    elseif h <= 20000
        T = 216.65;
        p = 22632.1*exp(-g0*(h - 11000)/(R*T));
        rho = p/(R*T);
    % Upper Stratosphere (20km to 32km)
    elseif h <= 32000
        T = 216.65 + 0.001*(h - 20000);
        p20 = 5474.889;
        p = p20*(T/216.65)^(-g0/(R*0.001));
        rho = p/(R*T);
    % Stratosphere Upper Bound
    else
        T = 228.65;
        p20 = 5474.889;
        T32 = 228.65;
        p32 = p20*(T32/216.65)^(-g0/(R*0.001));
        rho32 = p32/(R*T32);
        rho = rho32*exp(-g0*(h - 32000)/(R*T));
    end
end

== matlab function UpdatedIRECModel/apogeePredictor1 ==
  settings: updateMethod=DISCRETE
  data: vel input; p_curr input; thrust input; Cd_add_cmd output; tgt_p input; currentTime input; p_apogee_est output; t_apogee output; Cd_body input; mach input
function [Cd_add_cmd, p_apogee_est, t_apogee] = apogeePredictorPressure(vel, p_curr, thrust, tgt_p, currentTime, Cd_body, mach)
    persistent Cd_add_prev t_prev apogee_time prev_vel_up

    m = 18.9;
    A = 8107/(1000^2);
    A_over_m = A/m;
    g0 = 9.80665;
    Re = 6371000;

    Cd_body_nominal = 0.7;
    Cd_total_max = 1.7;

    if nargin < 6 || isempty(Cd_body)
        Cd_body = Cd_body_nominal;
    end
    if nargin < 7 || isempty(mach)
        mach = 0;
    end

    Cd_body = max(0, Cd_body);

    Cd_air_min = 0;
    Cd_air_max = max(0, Cd_total_max - Cd_body);

    burn_window = 3.0;
    thrust_thresh = 1.0;
    alt_tol = 0.0;
    max_iter = 12;
    max_rate = 1.5;

    if isempty(Cd_add_prev)
        Cd_add_prev = 0;
    end
    if isempty(t_prev)
        t_prev = currentTime;
    end
    if isempty(apogee_time)
        apogee_time = NaN;
    end
    if isempty(prev_vel_up)
        prev_vel_up = 0;
    end

    dt_cmd = currentTime - t_prev;
    if dt_cmd <= 0
        dt_cmd = 0.02;
    elseif dt_cmd > 0.1
        dt_cmd = 0.1;
    end
    t_prev = currentTime;

    Cd_add_prev = max(Cd_air_min, min(Cd_air_max, Cd_add_prev));

    alt_up = altFromPressure(p_curr, g0);

    if numel(vel) >= 3
        vel_up = -vel(3);
    else
        vel_up = vel;
    end

    thrust_mag = norm(thrust);

    if isnan(apogee_time)
        if prev_vel_up > 0 && vel_up <= 0
            apogee_time = currentTime;
        end
    end
    prev_vel_up = vel_up;

    tgt_alt = altFromPressure(tgt_p, g0);

    Cd_add_target = Cd_add_prev;
    apogee_est = alt_up;
    t_apogee = currentTime;
    p_apogee_est = p_curr;

    if ~isnan(apogee_time) && currentTime >= apogee_time + 2
        Cd_add_target = 0;
        apogee_est = alt_up;
        p_apogee_est = p_curr;
        t_apogee = apogee_time;

    elseif currentTime < burn_window && thrust_mag > thrust_thresh
        Cd_add_target = 0;

    elseif mach > 1
        Cd_add_target = 0;
        [apogee_est, dt_est] = simulateCoastVarCd(alt_up, vel_up, Cd_body, Cd_add_prev, Cd_add_target, max_rate, A_over_m, g0, Re);
        t_apogee = currentTime + dt_est;
        p_apogee_est = pressureAtAlt(apogee_est, g0);

    elseif vel_up <= 0
        Cd_add_target = Cd_air_max;
        [apogee_est, dt_est] = simulateCoastVarCd(alt_up, vel_up, Cd_body, Cd_add_prev, Cd_add_target, max_rate, A_over_m, g0, Re);
        t_apogee = currentTime + dt_est;
        p_apogee_est = pressureAtAlt(apogee_est, g0);

    elseif alt_up >= tgt_alt
        Cd_add_target = Cd_air_max;
        [apogee_est, dt_est] = simulateCoastVarCd(alt_up, vel_up, Cd_body, Cd_add_prev, Cd_add_target, max_rate, A_over_m, g0, Re);
        t_apogee = currentTime + dt_est;
        p_apogee_est = pressureAtAlt(apogee_est, g0);

    else
        [ap_clean, dt_clean] = simulateCoastVarCd(alt_up, vel_up, Cd_body, Cd_add_prev, 0, max_rate, A_over_m, g0, Re);

        if ap_clean <= tgt_alt + alt_tol
            Cd_add_target = 0;
            apogee_est = ap_clean;
            t_apogee = currentTime + dt_clean;
            p_apogee_est = pressureAtAlt(apogee_est, g0);

        elseif Cd_air_max <= 0
            Cd_add_target = 0;
            apogee_est = ap_clean;
            t_apogee = currentTime + dt_clean;
            p_apogee_est = pressureAtAlt(apogee_est, g0);

        else
            [ap_brake, dt_brake] = simulateCoastVarCd(alt_up, vel_up, Cd_body, Cd_add_prev, Cd_air_max, max_rate, A_over_m, g0, Re);

            if ap_brake > tgt_alt
                Cd_add_target = Cd_air_max;
                apogee_est = ap_brake;
                t_apogee = currentTime + dt_brake;
                p_apogee_est = pressureAtAlt(apogee_est, g0);
            else
                lowAdd = 0;
                highAdd = Cd_air_max;
                lowAp = ap_clean;
                highAp = ap_brake;
                lowT = dt_clean;
                highT = dt_brake;
                Cd_add_target = Cd_add_prev;

                for k = 1:max_iter
                    midAdd = 0.5*(lowAdd + highAdd);
                    [midAp, midT] = simulateCoastVarCd(alt_up, vel_up, Cd_body, Cd_add_prev, midAdd, max_rate, A_over_m, g0, Re);

                    if abs(midAp - tgt_alt) <= alt_tol
                        Cd_add_target = midAdd;
                        apogee_est = midAp;
                        t_apogee = currentTime + midT;
                        p_apogee_est = pressureAtAlt(apogee_est, g0);
                        break;
                    end

                    if midAp > tgt_alt
                        lowAdd = midAdd;
                        lowAp = midAp;
                        lowT = midT;
                    else
                        highAdd = midAdd;
                        highAp = midAp;
                        highT = midT;
                    end

                    if k == max_iter
                        Cd_add_target = 0.5*(lowAdd + highAdd);
                        [apogee_est, dt_final] = simulateCoastVarCd(alt_up, vel_up, Cd_body, Cd_add_prev, Cd_add_target, max_rate, A_over_m, g0, Re);
                        t_apogee = currentTime + dt_final;
                        p_apogee_est = pressureAtAlt(apogee_est, g0);
                    end
                end
            end
        end
    end

    Cd_add_target = max(Cd_air_min, min(Cd_air_max, Cd_add_target));

    max_step = max_rate * dt_cmd;
    delta = Cd_add_target - Cd_add_prev;
    if delta > max_step
        delta = max_step;
    elseif delta < -max_step
        delta = -max_step;
    end

    Cd_add_cmd = Cd_add_prev + delta;
    Cd_add_cmd = max(Cd_air_min, min(Cd_air_max, Cd_add_cmd));

    Cd_add_prev = Cd_add_cmd;
end

function [apogee, dt_to_apogee] = simulateCoastVarCd(h0, v0, Cd_body, Cd_add_initial, Cd_add_target, max_rate, A_over_m, g0, Re)
    if v0 <= 0
        apogee = max(0, h0);
        dt_to_apogee = 0;
        return;
    end

    h = h0;
    v = v0;
    t = 0;

    dt = 0.02;
    dt_min = 0.001;
    dt_max = 0.05;
    tol_h = 0.02;
    tol_v = 0.02;
    max_steps = 9000;

    Cd_add_initial = max(0, Cd_add_initial);
    Cd_add_target = max(0, Cd_add_target);

    for step = 1:max_steps
        while true
            [h_full, v_full] = rk4StepVarCd(h, v, t, dt, Cd_body, Cd_add_initial, Cd_add_target, max_rate, A_over_m, g0, Re);
            [h_half1, v_half1] = rk4StepVarCd(h, v, t, 0.5*dt, Cd_body, Cd_add_initial, Cd_add_target, max_rate, A_over_m, g0, Re);
            [h_half, v_half] = rk4StepVarCd(h_half1, v_half1, t + 0.5*dt, 0.5*dt, Cd_body, Cd_add_initial, Cd_add_target, max_rate, A_over_m, g0, Re);

            err_h = abs(h_half - h_full);
            err_v = abs(v_half - v_full);

            if err_h > tol_h || err_v > tol_v
                dt = max(dt_min, 0.5*dt);
                continue;
            end

            h_next = h_half;
            v_next = v_half;
            break;
        end

        if v > 0 && v_next <= 0
            Cd_add_now = cdProfile(t, Cd_add_initial, Cd_add_target, max_rate);
            Cd_total_now = Cd_body + Cd_add_now;
            a0 = computeAccel(h, v, Cd_total_now, A_over_m, g0, Re);
            frac = v/(v - v_next);
            t_zero = frac*dt;
            apogee = h + v*t_zero + 0.5*a0*t_zero^2;
            apogee = max(0, apogee);
            dt_to_apogee = t + t_zero;
            return;
        end

        h = h_next;
        v = v_next;
        t = t + dt;

        if err_h < 0.2*tol_h && err_v < 0.2*tol_v
            dt = min(dt_max, dt*1.25);
        end

        if h <= 0
            apogee = 0;
            dt_to_apogee = t;
            return;
        end
    end

    apogee = max(0, h);
    dt_to_apogee = t;
end

function [h_out, v_out] = rk4StepVarCd(h, v, t, dt, Cd_body, Cd_add_initial, Cd_add_target, max_rate, A_over_m, g0, Re)
    Cd_add1 = cdProfile(t, Cd_add_initial, Cd_add_target, max_rate);
    Cd_total1 = Cd_body + Cd_add1;
    k1_v = computeAccel(h, v, Cd_total1, A_over_m, g0, Re);
    k1_h = v;

    t2 = t + 0.5*dt;
    v2 = v + 0.5*dt*k1_v;
    h2 = h + 0.5*dt*k1_h;
    Cd_add2 = cdProfile(t2, Cd_add_initial, Cd_add_target, max_rate);
    Cd_total2 = Cd_body + Cd_add2;
    k2_v = computeAccel(h2, v2, Cd_total2, A_over_m, g0, Re);
    k2_h = v2;

    v3 = v + 0.5*dt*k2_v;
    h3 = h + 0.5*dt*k2_h;
    Cd_add3 = cdProfile(t2, Cd_add_initial, Cd_add_target, max_rate);
    Cd_total3 = Cd_body + Cd_add3;
    k3_v = computeAccel(h3, v3, Cd_total3, A_over_m, g0, Re);
    k3_h = v3;

    t4 = t + dt;
    v4 = v + dt*k3_v;
    h4 = h + dt*k3_h;
    Cd_add4 = cdProfile(t4, Cd_add_initial, Cd_add_target, max_rate);
    Cd_total4 = Cd_body + Cd_add4;
    k4_v = computeAccel(h4, v4, Cd_total4, A_over_m, g0, Re);
    k4_h = v4;

    v_out = v + (dt/6)*(k1_v + 2*k2_v + 2*k3_v + k4_v);
    h_out = h + (dt/6)*(k1_h + 2*k2_h + 2*k3_h + k4_h);
end

function Cd_add = cdProfile(t, Cd_initial, Cd_target, max_rate)
    delta = Cd_target - Cd_initial;
    max_delta = max_rate * t;

    if delta > 0
        delta_eff = min(delta, max_delta);
    else
        delta_eff = max(delta, -max_delta);
    end

    Cd_add = Cd_initial + delta_eff;
end

function a = computeAccel(h, v, Cd_total, A_over_m, g0, Re)
    rho = densityAtAlt(h, g0);
    g_eff = g0*(Re/(Re + h))^2;
    drag = -0.5*rho*Cd_total*A_over_m*v*abs(v);
    a = drag - g_eff;
end

function rho = densityAtAlt(h, g0)
    h = max(0, h);
    R = 287.053;
    if h <= 11000
        T = 288.15 - 0.0065*h;
        p = 101325*(T/288.15)^(g0/(R*0.0065));
        rho = p/(R*T);
    elseif h <= 20000
        T = 216.65;
        p = 22632.1*exp(-g0*(h - 11000)/(R*T));
        rho = p/(R*T);
    elseif h <= 32000
        T = 216.65 + 0.001*(h - 20000);
        p20 = 5474.889;
        p = p20*(T/216.65)^(-g0/(R*0.001));
        rho = p/(R*T);
    else
        T = 228.65;
        p20 = 5474.889;
        T32 = 228.65;
        p32 = p20*(T32/216.65)^(-g0/(R*0.001));
        rho32 = p32/(R*T32);
        rho = rho32*exp(-g0*(h - 32000)/(R*T));
    end
end

function h = altFromPressure(p, g0)
    p = max(min(p, 101325), 1);

    R = 287.053;
    p0 = 101325;
    T0 = 288.15;
    L1 = 0.0065;

    p11 = 22632.1;
    T11 = 216.65;

    p20 = 5474.889;
    T20 = 216.65;
    L2 = 0.001;

    T32 = 228.65;
    p32 = p20*(T32/T20)^(-g0/(R*L2));

    if p >= p11
        n1 = g0/(R*L1);
        T = T0*(p/p0)^(1/n1);
        h = (T0 - T)/L1;
    elseif p >= p20
        T = T11;
        h = 11000 - (R*T/g0)*log(p/p11);
    elseif p >= p32
        n2 = -g0/(R*L2);
        T = T20*(p/p20)^(1/n2);
        h = 20000 + (T - T20)/L2;
    else
        T = T32;
        h = 32000 - (R*T/g0)*log(p/p32);
    end

    h = max(0, h);
end

function p = pressureAtAlt(h, g0)
    h = max(0, h);
    R = 287.053;
    if h <= 11000
        T = 288.15 - 0.0065*h;
        p = 101325*(T/288.15)^(g0/(R*0.0065));
    elseif h <= 20000
        T = 216.65;
        p = 22632.1*exp(-g0*(h - 11000)/(R*T));
    elseif h <= 32000
        T = 216.65 + 0.001*(h - 20000);
        p20 = 5474.889;
        p = p20*(T/216.65)^(-g0/(R*0.001));
    else
        T = 228.65;
        p20 = 5474.889;
        T32 = 228.65;
        p32 = p20*(T32/216.65)^(-g0/(R*0.001));
        p = p32*exp(-g0*(h - 32000)/(R*T));
    end
end
